simulink model "TC_C0_ETH_PID"  (R2026a)
settings: Solver=ode1  EnableMultiTasking=on
model workspace (MAT data in the model file):
  K_cte_forward = 1
  K_cte_reverse = 0.25
  L_AXLE_DIST = 3
  MAX_STEERING_ANGLE_DEG = 35
undefined symbols (not defined in the file): TC_C0_ETH_PID
libraries: aurixtc4xxlib x8, simulink x3, AurixNetLib x3, procinterlib x2, aurixutilitieslib x2, slpidlib x1
settings Model: Creator=ttichy  LastModifiedBy=chmurski
settings SolverCC: PositivePriorityOrder=on
settings OptimizationCC: StrengthReduction=on  MaxStackSize=2048
settings HardwareCC: ProdLargestAtomicInteger=Long  ProdHWDeviceType=Infineon->TriCore  HardwareBoardFeatureSet=SoCBlockset
settings ModelReferenceCC: ModelReferenceNumInstancesAllowed=Single
settings SFSimCC: SimCustomHeaderCode="#include \"SmmReset.h\""  SimUserSources=SmmReset.c  SimUserIncludeDirs=./Reset
settings RTWCC: SystemTargetFile=ert.tlc  HardwareBoard=Infineon AURIX TC4x  TLCOptions=-aInlineSetEventsForThisBaseRateFcn=TLC_FALSE -aSuppressMultiTaskScheduler=TLC_FALSE -aRateBasedStepFcn=1  GenerateReport=on  CustomHeaderCode="#include \"SmmReset.h\""  Toolchain=TASKING SmartCode for TriCore  BuildConfiguration=Specify  IncludeHyperlinkInReport=on  LaunchReport=on  GenerateTraceInfo=on  GenerateTraceReport=on  GenerateTraceReportSl=on  GenerateTraceReportSf=on  GenerateTraceReportEml=on  GenerateCodeMetricsReport=on  Description=Embedded Coder
settings RTWCC: CustomInclude=|
  | ./Reset
  | ..\LanLib\middleware\lwip\src\include
  | ..\LanLib\middleware\lwip\src\include\lwip
  | ..\LanLib\middleware\lwip\src\include\lwip\prot
  | ..\LanLib\middleware\lwip\port\include
  | ..\LanLib\middleware\lwip
  | ..\LanLib\Components\phy
  | ..\LanLib\Components\phy\std
  | ..\LanLib\Components\phy\com
  | c:\Infineon\iLLD\TC4x\v2.3.0\TC49A\Src\Libraries\iLLD\TC49A\CpuGeneric\Geth\Eth
  | c:\Infineon\iLLD\TC4x\v2.3.0\TC49A\Src\Libraries\iLLD\TC49A\Tricore\Cpu\Std
  | c:\Infineon\iLLD\TC4x\v2.3.0\TC49A\Src\Libraries\iLLD\TC49A\CpuGeneric\Port\Std
  | ..\LanLib\Configurations
  | ..\TriCore\_ref\TC_C0_ETH_PID
  | ..\TomLib
  | ..\LanLib
  | ..\LanLib\Components
  | ..\LanLib\Components\phy
  | ..\LanLib\Board
  | ..\LanLib\Board\TC499A_TriBoard_STD_V11
  | c:\Infineon\iLLD\TC4x\v2.3.0\TC49A\Src\Libraries\iLLD\TC49A\CpuGeneric\Hsphy\Hsphy
  | ..\LanLib\middleware
  | ..\LanLib\middleware\lwip\src\include\netif
settings RTWCC: CustomSource=|
  | SmmReset.c
  | AurixNetLib.c
  | UDP_Setup_LWIP.c
  | led.c
  | serialio.c
  | board_std.c
  | IfxGeth_Phy_Rtl8201fi.c
  | ethernetif.c
  | ..\LanLib\middleware\lwip\src\core\def.c
  | ..\LanLib\middleware\lwip\src\core\init.c
  | ..\LanLib\middleware\lwip\src\core\ip.c
  | ..\LanLib\middleware\lwip\src\core\mem.c
  | ..\LanLib\middleware\lwip\src\core\memp.c
  | ..\LanLib\middleware\lwip\src\core\netif.c
  | ..\LanLib\middleware\lwip\src\core\pbuf.c
  | ..\LanLib\middleware\lwip\src\core\stats.c
  | ..\LanLib\middleware\lwip\src\core\sys.c
  | ..\LanLib\middleware\lwip\src\core\timeouts.c
  | ..\LanLib\middleware\lwip\src\core\udp.c
  | ..\LanLib\middleware\lwip\src\core\inet_chksum.c
  | ..\LanLib\middleware\lwip\src\core\ipv4\etharp.c
  | ..\LanLib\middleware\lwip\src\core\ipv4\ip4.c
  | ..\LanLib\middleware\lwip\src\core\ipv4\ip4_addr.c
  | ..\LanLib\middleware\lwip\src\core\ipv4\ip4_frag.c
  | ..\LanLib\middleware\lwip\src\netif\ethernet.c
  | ..\LanLib\middleware\lwip\port\sys\sys_arch_nosys.c
  | ..\LanLib\middleware\lwip\src\core\ipv4\icmp.c
settings CodeAppCC: MaxIdLength=256.0
settings ERTTargetCC: ExtModeTransport=3.0  ERTFilePackagingFormat=Compact  DynamicArrayContainerType=coder::array  SupportAbsoluteTime=off  SupportNonFinite=off

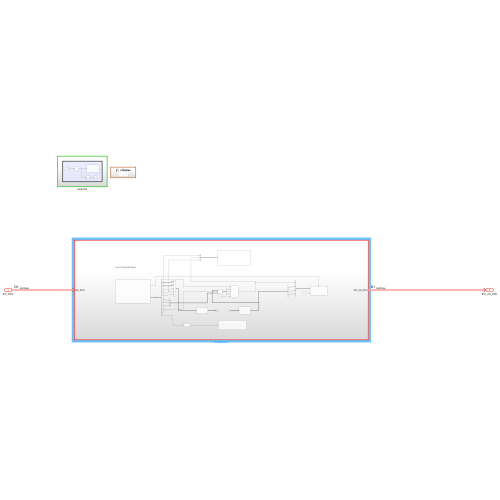
[thumbnail: Simulink's stored preview of the top-level diagram]
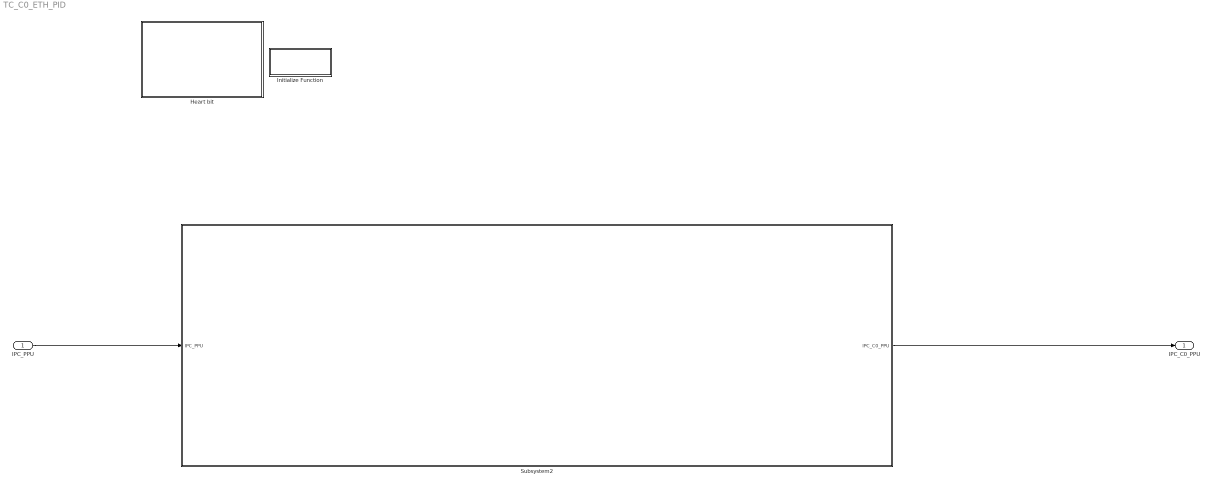
== system TC_C0_ETH_PID ==
  IPC_PPU : Inport  OutputPortMessageModes=m
  Heart bit : Subsystem  TreatAsAtomicUnit=on  SystemSampleTime=0.1
  Initialize Function : Subsystem  TreatAsAtomicUnit=on
  Subsystem2 : Subsystem  TreatAsAtomicUnit=on  SystemSampleTime=0.01
  IPC_C0_PPU : Outport  InputPortMessageModes=m
  wires:
  Subsystem2/1(IPC_C0_PPU) -> IPC_C0_PPU/1
  IPC_PPU/1 -> Subsystem2/1(IPC_PPU)

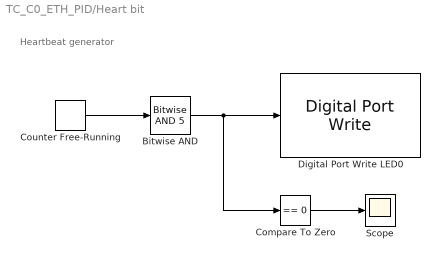
== system TC_C0_ETH_PID/Heart bit ==
  note: Heartbeat generator
  Bitwise AND : simulink/Logic and Bit Operations/Bitwise Operator  logicop=AND  UseBitMask=on  BitMask=5  BitMaskRealWorld=Stored Integer
      settings: LibrarySourceBlock=|
      | simulink/Quick Insert/Logic and Bit
      | Operations/Bitwise AND
  Compare To Zero : simulink/Logic and Bit Operations/Compare To Zero  relop===  OutDataTypeStr=boolean
  Counter Free-Running : simulink/Sources/Counter Free-Running  NumBits=32  tsamp=.1
  Digital Port Write LED0 : aurixtc4xxlib/Digital Port Write  numPins=1  BlockSID=TC_C0_ETH_PID:4  PeripheralConfigBtnCtrl=0  enableSimPort=off  simMode=SoC Data (Message based)
  Scope : Scope
      settings: ActiveDisplayYMinimum=-0.125  ActiveDisplayYMaximum=1.125
  wires:
  Bitwise AND/1 -> Compare To Zero/1, Digital Port Write LED0/1
  Compare To Zero/1 -> Scope/1
  Counter Free-Running/1 -> Bitwise AND/1

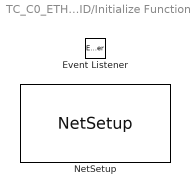
== system TC_C0_ETH_PID/Initialize Function ==
  Event Listener : EventListener  DisableCoverage=on  EventName=reset
  NetSetup : AurixNetLib/NetSetup  ip=[192,168,178,5]  netmask=[255,255,255,0]  gw=[192,168,178,1]  SampleTime=-1

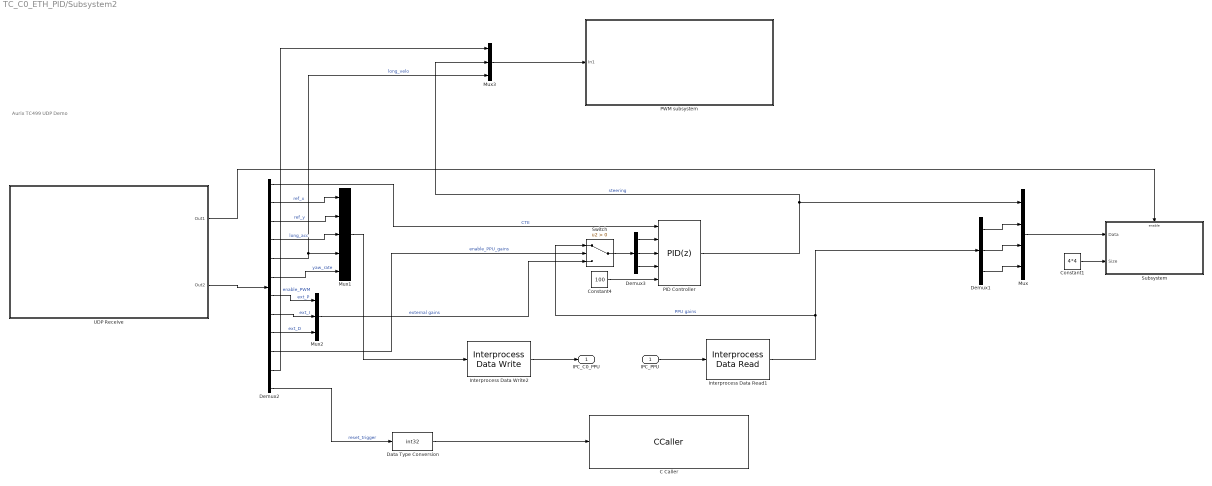
== system TC_C0_ETH_PID/Subsystem2 ==
  note: Aurix TC499 UDP Demo
  IPC_PPU : Inport
  C Caller : CCaller  FunctionName=SmmReset_triggerReset  PortSpecificationStruct="%)30     .    * (   8    (     @         %    \"     $    !     0         %  0 \"0    $    _    07)G3F%M90  4&]R=$YA;64 4V-O<&4     26YD97@     5'EP90      4VEZ90      27-';&]B86P   X    X    !@    @    $          4    (     0    8    !         !     &    96YA8FQE   .    .     8    (    !          %    \"     $    &     0         0    !@   &5N86)L90  #@   #@    &    \"     0         !0    @    !    !0    $         $     4   !);G!U=     X    X    !@    @    &          4    (     0    $    !          D    (               .    .     8    (    !          %    \"     $    %     0         0    !0   &EN=#,R    #@   #     &    \"     0         !0    @    !     0    $         $  ! #$    .    ,     8    (    \"0(        %    \"     $    !     0         \"  $"
  Constant1 : Constant  Value=4*4  OutDataTypeStr=uint16
  Constant4 : Constant  Value=100  OutDataTypeStr=single
  Data Type Conversion : DataTypeConversion  OutDataTypeStr=int32  SaturateOnIntegerOverflow=off  RndMeth=Floor
  Demux1 : Demux  Outputs=[1,1,1]
  Demux2 : Demux  Outputs=[1,5,5,1,1,1,1,1,1,1,1,1]
  Demux3 : Demux  Outputs=[1,1,1]
  Interprocess Data Read1 : procinterlib/Interprocess Data Read  showPort=on  DataType=single  NumBuffers=1  DataLength=3  ChannelNum=1  IsIntEnabled=0  EnInterrupt=off  StructForBus=struct( 'signal1', uint16( 0 ), 'signal2', uint16( 0 ) )  IPCBetween=5  CurrentPU=0  PartCores=TriCore0<->PPU  SampleTime=-1  TargetType=1  ClientPU=PPU  ClientIntPrio=45  CurrentPUPriority=0
  Interprocess Data Write2 : procinterlib/Interprocess Data Write  showPort=on  ChannelNum=0  NumBuff=1  IsIntEnabled=1  EnInterrupt=off  IPCBetween=5  CurrentPU=0  DataType=single  PartCores=TriCore0<->PPU  TargetType=1  ClientPU=PPU  ClientIntPrio=50  CurrentPUPriority=0
      settings: LibrarySourceBlock=c2000lib/Target Communication/Interprocess Data Write
  Mux : Mux
  Mux1 : Mux  Inputs=5
  Mux2 : Mux  Inputs=3
  Mux3 : Mux  Inputs=3
  PID Controller : slpidlib/PID Controller  Controller=PID  Form=Parallel  TimeDomain=Discrete-time  UseExternalTs=off  SampleTime=-1  IntegratorMethod=Forward Euler  FilterMethod=Forward Euler  ControllerParametersSource=external  P=1  I=1  UseKiTs=on  D=0  UseExternalDerivativeSource=off  N=100  UseFilter=on  TunerSelectOption=Transfer Function Based (PID Tuner App)  InitialConditionSource=internal  InitialConditionForIntegrator=0  InitialConditionForFilter=0  DifferentiatorICPrevScaledInput=0  ExternalReset=none  TrackingMode=off  Kt=1  LimitOutput=on  SatLimitsSource=internal  UpperSaturationLimit=35  LowerSaturationLimit=-35  LinearizeAsGain=on  AntiWindupMode=back-calculation  Kb=10  LimitIntegrator=off  UpperIntegratorSaturationLimit=inf  LowerIntegratorSaturationLimit=-inf  POutMin=[]  POutMax=[]  IOutMin=[]  IOutMax=[]  DOutMin=[]  DOutMax=[]  NOutMin=[]  NOutMax=[]  SumOutMin=[]  SumOutMax=[]  SaturationOutMin=[]  SaturationOutMax=[]  PParamMin=[]  PParamMax=[]  IParamMin=[]  IParamMax=[]  DParamMin=[]  DParamMax=[]  NParamMin=[]  NParamMax=[]  KbParamMin=[]  KbParamMax=[]  KtParamMin=[]  KtParamMax=[]  KbOutMin=[]  KbOutMax=[]  KtOutMin=[]  KtOutMax=[]  IntegratorOutMin=[]  IntegratorOutMax=[]  FilterOutMin=[]  FilterOutMax=[]  SumI1OutMin=[]  SumI1OutMax=[]  SumI2OutMin=[]  SumI2OutMax=[]  SumI3OutMin=[]  SumI3OutMax=[]  SumI4OutMin=[]  SumI4OutMax=[]  SumDOutMin=[]  SumDOutMax=[]  DifferentiatorOutMin=[]  DifferentiatorOutMax=[]  FilterDiffOutCoefMin=[]  FilterDiffOutCoefMax=[]  ReciprocalOutMin=[]  ReciprocalOutMax=[]  SumDenOutMin=[]  SumDenOutMax=[]  SumNumOutMin=[]  SumNumOutMax=[]  DivideOutMin=[]  DivideOutMax=[]  UdiffTsProdOutMin=[]  UdiffTsProdOutMax=[]  NTsProdOutMin=[]  NTsProdOutMax=[]  UintegralTsProdOutMin=[]  UintegralTsProdOutMax=[]  UngainTsProdOutMin=[]  UngainTsProdOutMax=[]  ClampingZeroOutDataTypeStr=Inherit: Inherit via back propagation  ClampingZeroOutMin=[]  ClampingZeroOutMax=[]  FilterDenConstantOutDataTypeStr=Inherit: Inherit via back propagation  FilterDenConstantOutMin=[]  FilterDenConstantOutMax=[]  PCopyOutDataTypeStr=Inherit: Inherit via back propagation  PCopyOutMin=[]  PCopyOutMax=[]  NCopyOutDataTypeStr=Inherit: Inherit via back propagation  NCopyOutMin=[]  NCopyOutMax=[]  IntegratorContinuousStateAttributes=''  IntegratorStateMustResolveToSignalObject=off  IntegratorRTWStateStorageClass=Auto  FilterContinuousStateAttributes=''  FilterStateMustResolveToSignalObject=off  FilterRTWStateStorageClass=Auto  ParallelPVariant=ExternalParameters  IdealPVariant=Disabled  IVariant=ExternalParameters  DVariant=ExternalParameters  IntegratorVariant=Discrete  SatVariant=Enabled  AWVariant=BackCalculation  PCopyVariant=Disabled  TRVariant=Disabled  FdbkBlocksVariant=Forward  IdealPFdbkVariant=Disabled  SatFdbkVariant=Disabled  DerivativeFilterVariant=ForwardEulerFilter  NVariant=ExternalParameters  NCopyVariant=Disabled  FilterICVariant=InternalICsFilter  IntegratorICVariant=InternalICs  ExternalResetVariant=Disabled  TRSumVariant=Passthrough  SumFdbkVariant=Disabled  SumVariant=Sum_PID  TsampFilterVariant=InternalTs  TsampNgainVariant=Passthrough  TsampIntegralVariant=Disabled_SignalSpec  ExternalSaturationOutDataTypeStr=Inherit: Same as second input  DerivativeSourceVariant=ErrorSignal  PreIntVariant=InternalPreInt
  PWM subsystem : Subsystem
  Subsystem : Subsystem
  Switch : Switch  Criteria=u2 > Threshold  SaturateOnIntegerOverflow=off  InputSameDT=off
  UDP Receive : Subsystem
  IPC_C0_PPU : Outport
  wires:
  Mux/1 -> Subsystem/1(Data)
  Interprocess Data Write2/1 -> IPC_C0_PPU/1
  Constant1/1 -> Subsystem/2(Size)
  UDP Receive/2(Out2) -> Demux2/1
  UDP Receive/1(Out1) -> Subsystem/Enable
  IPC_PPU/1 -> Interprocess Data Read1/1
  Interprocess Data Read1/1 -> Switch/1, Demux1/1  "PPU gains"
  PID Controller/1 -> Mux3/2, Mux/1  "steering"
  Demux3/2 -> PID Controller/3
  Demux3/1 -> PID Controller/2
  Constant4/1 -> PID Controller/5
  Demux3/3 -> PID Controller/4
  Demux2/1 -> PID Controller/1  "CTE"
  Demux2/2 -> Mux1/1  "ref_x"
  Demux2/3 -> Mux1/2  "ref_y"
  Demux2/4 -> Mux1/3  "long_acc"
  Demux2/5 -> Mux1/4, Mux3/3  "long_velo"
  Demux2/7 -> Mux2/1  "ext_P"
  Demux2/8 -> Mux2/2  "ext_I"
  Demux2/9 -> Mux2/3  "ext_D"
  Demux2/10 -> Switch/2  "enable_PPU_gains"
  Mux1/1 -> Interprocess Data Write2/1
  Switch/1 -> Demux3/1
  Mux2/1 -> Switch/3  "external gains"
  Mux3/1 -> PWM subsystem/1(In1)
  Demux2/11 -> Mux3/1  "enable_PWM"
  Demux2/12 -> Data Type Conversion/1  "reset_trigger"
  Data Type Conversion/1 -> C Caller/1
  Demux2/6 -> Mux1/5  "yaw_rate"
  Demux1/1 -> Mux/2
  Demux1/2 -> Mux/3
  Demux1/3 -> Mux/4

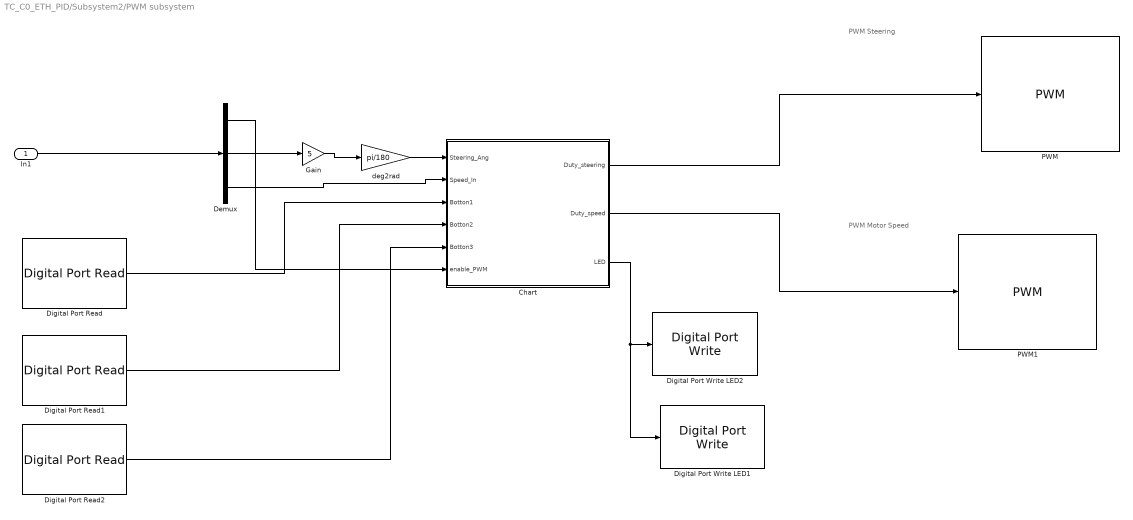
== system TC_C0_ETH_PID/Subsystem2/PWM subsystem ==
  note: PWM Motor Speed
  note: PWM Steering
  In1 : Inport
  Chart : Stateflow chart  TreatAsAtomicUnit=on
  Demux : Demux  Outputs=3
  Digital Port Read : aurixtc4xxlib/Digital Port Read  numPins=1  SampleTime=-1  BlockSID=TC_C0_ETH_PID:258  PeripheralConfigBtnCtrl=0  enableSimPort=off  simMode=SoC Data (Message based)
  Digital Port Read1 : aurixtc4xxlib/Digital Port Read  numPins=1  SampleTime=-1  BlockSID=TC_C0_ETH_PID:259  PeripheralConfigBtnCtrl=0  enableSimPort=off  simMode=SoC Data (Message based)
  Digital Port Read2 : aurixtc4xxlib/Digital Port Read  numPins=1  SampleTime=-1  BlockSID=TC_C0_ETH_PID:260  PeripheralConfigBtnCtrl=0  enableSimPort=off  simMode=SoC Data (Message based)
  Digital Port Write LED1 : aurixtc4xxlib/Digital Port Write  numPins=1  BlockSID=TC_C0_ETH_PID:262  PeripheralConfigBtnCtrl=0  enableSimPort=off  simMode=SoC Data (Message based)
  Digital Port Write LED2 : aurixtc4xxlib/Digital Port Write  numPins=1  BlockSID=TC_C0_ETH_PID:263  PeripheralConfigBtnCtrl=0  enableSimPort=off  simMode=SoC Data (Message based)
  Gain : Gain  Gain=5
  PWM : aurixtc4xxlib/PWM  enableFreq=off  enablePhase=off  PeripheralConfigBtnCtrl=0  enableStatus=off  BlockSID=TC_C0_ETH_PID:264  enableSimPort=off  simMode=SoC Data (Message based)  numChannel=1  enableDTM=off
  PWM1 : aurixtc4xxlib/PWM  enableFreq=off  enablePhase=off  PeripheralConfigBtnCtrl=0  enableStatus=off  BlockSID=TC_C0_ETH_PID:265  enableSimPort=off  simMode=SoC Data (Message based)  numChannel=1  enableDTM=off
  deg2rad : Gain  Gain=pi/180
  wires:
  In1/1 -> Demux/1
  Chart/1(Duty_steering) -> PWM/1
  Chart/3(LED) -> Digital Port Write LED2/1, Digital Port Write LED1/1
  Digital Port Read2/1 -> Chart/5(Botton3)
  Demux/1 -> Chart/6(enable_PWM)
  Chart/2(Duty_speed) -> PWM1/1
  Demux/2 -> Gain/1
  Digital Port Read1/1 -> Chart/4(Botton2)
  Digital Port Read/1 -> Chart/3(Botton1)
  Demux/3 -> Chart/2(Speed_In)
  deg2rad/1 -> Chart/1(Steering_Ang)
  Gain/1 -> deg2rad/1

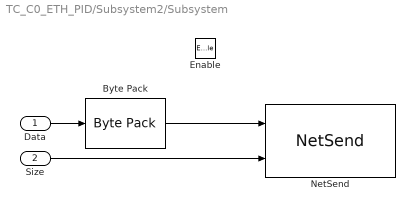
== system TC_C0_ETH_PID/Subsystem2/Subsystem ==
  Data : Inport
  Size : Inport  Port=2
  Enable : EnablePort
  Byte Pack : aurixutilitieslib/Byte Pack  datatypes={'single'}  byteAlign=1  blockPlatform=stm32f4discovery
  NetSend : AurixNetLib/NetSend  SampleTime=0.01
  wires:
  Size/1 -> NetSend/2
  Data/1 -> Byte Pack/1
  Byte Pack/1 -> NetSend/1

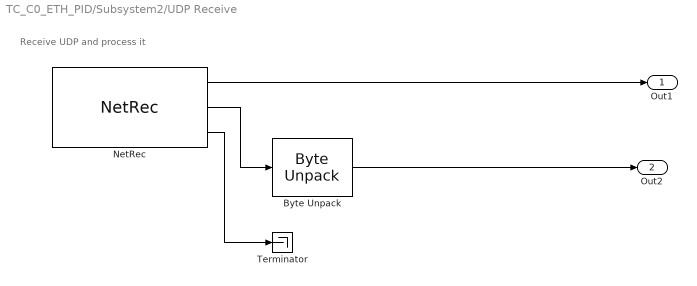
== system TC_C0_ETH_PID/Subsystem2/UDP Receive ==
  note: Receive UDP and process it
  Byte Unpack : aurixutilitieslib/Byte Unpack  dimensions={[20]}  datatypes={'single'}  byteAlign=1  blockPlatform=stm32f4discovery
  NetRec : AurixNetLib/NetRec  maxSize=20*4  SampleTime=0.01
  Terminator : Terminator
  Out1 : Outport
  Out2 : Outport  Port=2
  wires:
  NetRec/3 -> Terminator/1
  NetRec/2 -> Byte Unpack/1
  Byte Unpack/1 -> Out2/1
  NetRec/1 -> Out1/1

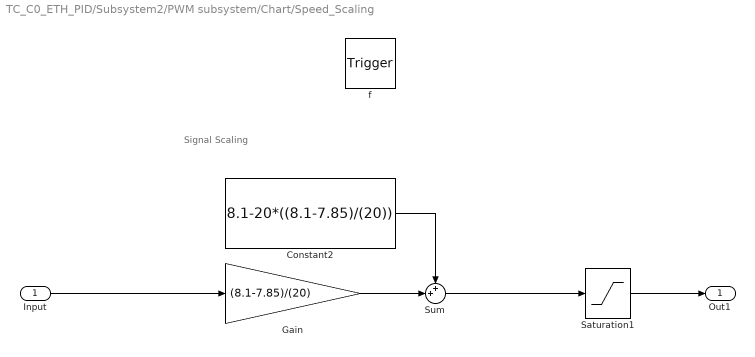
== system TC_C0_ETH_PID/Subsystem2/PWM subsystem/Chart/Speed_Scaling ==
  note: Signal Scaling
  Input : Inport  OutDataTypeStr=single  PortDimensions=1
  f : TriggerPort  TriggerType=function-call  VariantControl=(inherit)
      settings: CopyFcn=Stateflow.SLINSF.SimulinkMan.removeBlockPreDeleteFcn  PreDeleteFcn=Stateflow.SLINSF.SimulinkMan.unsafePredeleteFcn
  Constant2 : Constant  Value=8.1-20*((8.1-7.85)/(20))  OutDataTypeStr=single
  Gain : Gain  Gain=(8.1-7.85)/(20)
  Saturation1 : Saturate  UpperLimit=8  LowerLimit=7.9
      settings: LockScale=on
  Sum : Sum  Inputs=++|
  Out1 : Outport  OutDataTypeStr=single
  wires:
  Sum/1 -> Saturation1/1
  Saturation1/1 -> Out1/1
  Constant2/1 -> Sum/1
  Input/1 -> Gain/1
  Gain/1 -> Sum/2

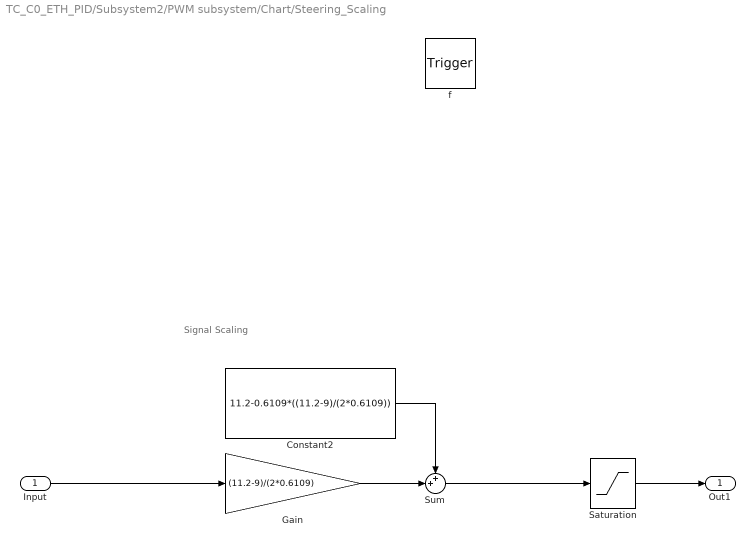
== system TC_C0_ETH_PID/Subsystem2/PWM subsystem/Chart/Steering_Scaling ==
  note: Signal Scaling
  Input : Inport  OutDataTypeStr=single  PortDimensions=1
  f : TriggerPort  TriggerType=function-call  VariantControl=(inherit)
      settings: CopyFcn=Stateflow.SLINSF.SimulinkMan.removeBlockPreDeleteFcn  PreDeleteFcn=Stateflow.SLINSF.SimulinkMan.unsafePredeleteFcn
  Constant2 : Constant  Value=11.2-0.6109*((11.2-9)/(2*0.6109))  OutDataTypeStr=single
  Gain : Gain  Gain=(11.2-9)/(2*0.6109)
  Saturation : Saturate  UpperLimit=11.2  LowerLimit=9
  Sum : Sum  Inputs=++|
  Out1 : Outport  OutDataTypeStr=single
  wires:
  Constant2/1 -> Sum/1
  Gain/1 -> Sum/2
  Input/1 -> Gain/1
  Sum/1 -> Saturation/1
  Saturation/1 -> Out1/1

== stateflow chart TC_C0_ETH_PID/Subsystem2/PWM subsystem/Chart ==
  state Calibration
    Duty_steering = 10.2;
    Duty_speed = 7.5;
    LED = 0; % Off
  state Operation_Duty
    Duty_steering = Steering_Scaling(Steering_Ang);
    Duty_speed = Speed_Scaling(Speed_In);
    LED = 1; % On
  state Out1 = Steering_Scaling(Input) [function]
  state Out1 = Speed_Scaling(Input) [function]
  (default) -> Calibration
  Calibration -> Operation_Duty : [enable_PWM >= 1&&Speed_In >0]
  Operation_Duty -> Calibration : [enable_PWM <=0 || Speed_In <=0 ]
  data: Input function_input single size=1; Out1 function_output single; Input function_input single size=1; Out1 function_output single; Steering_Ang input single; Speed_In input single; Botton1 input boolean; Botton2 input boolean; Botton3 input boolean; Duty_steering output single; Duty_speed output single; LED output; enable_PWM input single
